simulink model "usato"  (R2016a)
settings: Solver=ode3  StartTime=0.0  StopTime=200  FixedStep=0.1  RelTol=1e-5
values from neighbouring files (symbols this model uses):
  c = 0.1    [Script.m]
  Kd = 0.9    [Script.m]
  Ki = 0.036    [Script.m]
  Kp = 0.37    [Script.m]
  N = 5    [Script.m]
libraries: simulink x2
(part 2 of 2)

== matlab function usato/sigma2 pi5 ==
  data: qpi_d_k05 input; qpi_d_k05sigma output; C2k05 input
function qpi_d_k05sigma=sigma(qpi_d_k05,C2k05)
    if(qpi_d_k05 > C2k05)
        qpi_d_k05sigma=C2k05;
    
    else
        if(qpi_d_k05 < -C2k05)
            qpi_d_k05sigma =-C2k05;
        else
        if(qpi_d_k05 == 0)
                qpi_d_k05sigma=0;
        else
            qpi_d_k05sigma=qpi_d_k05;
        end
        end
    end

== matlab function usato/sigma1 pi6 ==
  data: qpi_k02 input; qpi_k02sigma output
function qpi_k02sigma=sigma(qpi_k02)
    if(qpi_k02 > 1.05)
        qpi_k02sigma=1.05;
    
    else
        if(qpi_k02 < -1.05)
            qpi_k02sigma = -1.05;
        else
        if(qpi_k02 == 0)
                qpi_k02sigma=0;
        else
            qpi_k02sigma=qpi_k02;
        end
        end
    end

== matlab function usato/sigma2 pi6 ==
  data: qpi_d_k02 input; qpi_d_k02sigma output; C2k02 input
function qpi_d_k02sigma=sigma(qpi_d_k02,C2k02)
    if(qpi_d_k02 > C2k02)
        qpi_d_k02sigma=C2k02;
    
    else
        if(qpi_d_k02 < -C2k02)
            qpi_d_k02sigma =-C2k02;
        else
        if(qpi_d_k02 == 0)
                qpi_d_k02sigma=0;
        else
            qpi_d_k02sigma=qpi_d_k02;
        end
        end
    end

== matlab function usato/sigma1 pi7 ==
  data: qpi_k075 input; qpi_k075sigma output
function qpi_k075sigma=sigma(qpi_k075)
    if(qpi_k075 > 1.05)
        qpi_k075sigma=1.05;
    
    else
        if(qpi_k075 < -1.05)
            qpi_k075sigma = -1.05;
        else
        if(qpi_k075 == 0)
                qpi_k075sigma=0;
        else
            qpi_k075sigma=qpi_k075;
        end
        end
    end

== matlab function usato/sigma2 pi7 ==
  data: qpi_d_k075 input; qpi_d_k075sigma output; C2k075 input
function qpi_d_k075sigma=sigma(qpi_d_k075,C2k075)
    if(qpi_d_k075 > C2k075)
        qpi_d_k075sigma=C2k075;
    
    else
        if(qpi_d_k075 < -C2k075)
            qpi_d_k075sigma =-C2k075;
        else
        if(qpi_d_k075 == 0)
                qpi_d_k075sigma=0;
        else
            qpi_d_k075sigma=qpi_d_k075;
        end
        end
    end

== matlab function usato/MATLAB Function6 ==
  data: qpk01 input; qpk01sigma output
function qpk01sigma=sigma(qpk01)
    if(qpk01 > 1.05)
        qpk01sigma=1.05;
    
    else
        if(qpk01 < -1.05)
            qpk01sigma = -1.05;
        else
        if(qpk01 == 0)
                qpk01sigma=0;
        else
            qpk01sigma=qpk01;
        end
        end
    end

== matlab function usato/MATLAB Function7 ==
  data: qdk01 input; qdk01sigma output; c3pk01 input
function qdk01sigma=sigma(qdk01,c3pk01)

    if(qdk01 > c3pk01)
        qdk01sigma=c3pk01;
    
    else
        if(qdk01 < -c3pk01)
            qdk01sigma = -c3pk01;
        else
        if(qdk01 == 0)
                qdk01sigma=0;
        else
            qdk01sigma=qdk01;
        end
        end
    end

== matlab function usato/MATLAB Function8 ==
  data: qik01 input; qik01sigma output; c2pk01 input
function qik01sigma=sigma(qik01,c2pk01)
    if(qik01 > c2pk01)
        qik01sigma=c2pk01;
    
    else
        if(qik01 < -c2pk01)
            qik01sigma = -c2pk01;
        else
        if(qik01 == 0)
                qik01sigma=0;
        else
            qik01sigma=qik01;
        end
        end
    end

== matlab function usato/MATLAB Function10 ==
  data: qdk02 input; qdk02sigma output; C3pk02 input
function qdk02sigma=sigma(qdk02,C3pk02)

    if(qdk02 > C3pk02)
        qdk02sigma=C3pk02;
    
    else
        if(qdk02 < -C3pk02)
            qdk02sigma = -C3pk02;
        else
        if(qdk02 == 0)
                qdk02sigma=0;
        else
            qdk02sigma=qdk02;
        end
        end
    end

== matlab function usato/MATLAB Function11 ==
  data: qik02 input; qik02sigma output; C2pk02 input
function qik02sigma=sigma(qik02,C2pk02)
    if(qik02 > C2pk02)
        qik02sigma=C2pk02;
    
    else
        if(qik02 < -C2pk02)
            qik02sigma = -C2pk02;
        else
        if(qik02 == 0)
                qik02sigma=0;
        else
            qik02sigma=qik02;
        end
        end
    end

== matlab function usato/MATLAB Function9 ==
  data: qpk02 input; qpk02sigma output
function qpk02sigma=sigma(qpk02)
    if(qpk02 > 1.05)
        qpk02sigma=1.05;
    
    else
        if(qpk02 < -1.05)
            qpk02sigma = -1.05;
        else
        if(qpk02 == 0)
                qpk02sigma=0;
        else
            qpk02sigma=qpk02;
        end
        end
    end

== matlab function usato/MATLAB Function12 ==
  data: qdk05 input; qdk05sigma output; C3pk05 input
function qdk05sigma=sigma(qdk05,C3pk05)

    if(qdk05 > C3pk05)
        qdk05sigma=C3pk05;
    
    else
        if(qdk05 < -C3pk05)
            qdk05sigma = -C3pk05;
        else
        if(qdk05 == 0)
                qdk05sigma=0;
        else
            qdk05sigma=qdk05;
        end
        end
    end

== matlab function usato/MATLAB Function13 ==
  data: qik05 input; qik05sigma output; C2pk05 input
function qik05sigma=sigma(qik05,C2pk05)
    if(qik05 > C2pk05)
        qik05sigma=C2pk05;
    
    else
        if(qik05 < -C2pk05)
            qik05sigma = -C2pk05;
        else
        if(qik05 == 0)
                qik05sigma=0;
        else
            qik05sigma=qik05;
        end
        end
    end

== matlab function usato/MATLAB Function14 ==
  data: qpk05 input; qpk05sigma output
function qpk05sigma=sigma(qpk05)
    if(qpk05 > 1.05)
        qpk05sigma=1.05;
    
    else
        if(qpk05 < -1.05)
            qpk05sigma = -1.05;
        else
        if(qpk05 == 0)
                qpk05sigma=0;
        else
            qpk05sigma=qpk05;
        end
        end
    end

== matlab function usato/MATLAB Function15 ==
  data: qdk2 input; qdk2sigma output; C3pk2 input
function qdk2sigma=sigma(qdk2,C3pk2)

    if(qdk2 > C3pk2)
        qdk2sigma=C3pk2;
    
    else
        if(qdk2 < -C3pk2)
            qdk2sigma = -C3pk2;
        else
        if(qdk2 == 0)
                qdk2sigma=0;
        else
            qdk2sigma=qdk2;
        end
        end
    end

== matlab function usato/MATLAB Function16 ==
  data: qik2 input; qik2sigma output; C2pk2 input
function qik2sigma=sigma(qik2,C2pk2)
    if(qik2 > C2pk2)
        qik2sigma=C2pk2;
    
    else
        if(qik2 < -C2pk2)
            qik2sigma = -C2pk2;
        else
        if(qik2 == 0)
                qik2sigma=0;
        else
            qik2sigma=qik2;
        end
        end
    end

== matlab function usato/MATLAB Function17 ==
  data: qpk2 input; qpk2sigma output
function qpk2sigma=sigma(qpk2)
    if(qpk2 > 1.05)
        qpk2sigma=1.05;
    
    else
        if(qpk2 < -1.05)
            qpk2sigma = -1.05;
        else
        if(qpk2 == 0)
                qpk2sigma=0;
        else
            qpk2sigma=qpk2;
        end
        end
    end

== matlab function usato/MATLAB Function18 ==
  data: qdk26 input; qdk26sigma output; C3pk26 input
function qdk26sigma=sigma(qdk26,C3pk26)

    if(qdk26 > C3pk26)
        qdk26sigma=C3pk26;
    
    else
        if(qdk26 < -C3pk26)
            qdk26sigma = -C3pk26;
        else
        if(qdk26 == 0)
                qdk26sigma=0;
        else
            qdk26sigma=qdk26;
        end
        end
    end

== matlab function usato/MATLAB Function19 ==
  data: qik26 input; qik26sigma output; C2pk26 input
function qik26sigma=sigma(qik26,C2pk26)
    if(qik26 > C2pk26)
        qik26sigma=C2pk26;
    
    else
        if(qik26 < -C2pk26)
            qik26sigma = -C2pk26;
        else
        if(qik26 == 0)
                qik26sigma=0;
        else
            qik26sigma=qik26;
        end
        end
    end

== matlab function usato/MATLAB Function20 ==
  data: qpk26 input; qpk26sigma output
function qpk26sigma=sigma(qpk26)
    if(qpk26 > 1.05)
        qpk26sigma=1.05;
    
    else
        if(qpk26 < -1.05)
            qpk26sigma = -1.05;
        else
        if(qpk26 == 0)
                qpk26sigma=0;
        else
            qpk26sigma=qpk26;
        end
        end
    end

== matlab function usato/sigma1 pd1 ==
  data: qpd01 input; qpd01sigma output
function qpd01sigma=sigma(qpd01)
    if(qpd01 > 1.05)
        qpd01sigma=1.05;
    
    else
        if(qpd01 < -1.05)
            qpd01sigma = -1.05;
        else
        if(qpd01 == 0)
                qpd01sigma=0;
        else
            qpd01sigma=qpd01;
        end
        end
    end

== matlab function usato/sigma2 pd1 ==
  data: qi01 input; qi01sigma output; C2pd01 input
function qi01sigma=sigma(qi01,C2pd01)
    if(qi01 > C2pd01)
        qi01sigma=C2pd01;
    
    else
        if(qi01 < -C2pd01)
            qi01sigma = -C2pd01;
        else
        if(qi01 == 0)
                qi01sigma=0;
        else
            qi01sigma=qi01;
        end
        end
    end

== matlab function usato/sigma1 pd2 ==
  data: qpd001 input; qpd001sigma output
function qpd001sigma=sigma(qpd001)
    if(qpd001 > 1.05)
        qpd001sigma=1.05;
    
    else
        if(qpd001 < -1.05)
            qpd001sigma = -1.05;
        else
        if(qpd001 == 0)
                qpd001sigma=0;
        else
            qpd001sigma=qpd001;
        end
        end
    end

== matlab function usato/sigma2 pd2 ==
  data: qi001 input; qi001sigma output; C2pd001 input
function qi001sigma=sigma(qi001,C2pd001)
    if(qi001 > C2pd001)
        qi001sigma=C2pd001;
    
    else
        if(qi001 < -C2pd001)
            qi001sigma = -C2pd001;
        else
        if(qi001 == 0)
                qi001sigma=0;
        else
            qi001sigma=qi001;
        end
        end
    end

== matlab function usato/sigma1 pd3 ==
  data: qpd10 input; qpd10sigma output
function qpd10sigma=sigma(qpd10)
    if(qpd10 > 1.05)
        qpd10sigma=1.05;
    
    else
        if(qpd10 < -1.05)
            qpd10sigma = -1.05;
        else
        if(qpd10 == 0)
                qpd10sigma=0;
        else
            qpd10sigma=qpd10;
        end
        end
    end

== matlab function usato/sigma2 pd3 ==
  data: qi10 input; qi10sigma output; C2pd10 input
function qi10sigma=sigma(qi10,C2pd10)
    if(qi10 > C2pd10)
        qi10sigma=C2pd10;
    
    else
        if(qi10 < -C2pd10)
            qi10sigma = -C2pd10;
        else
        if(qi10 == 0)
                qi10sigma=0;
        else
            qi10sigma=qi10;
        end
        end
    end

== matlab function usato/sigma1 pd4 ==
  data: qpd0001 input; qpd0001sigma output
function qpd0001sigma=sigma(qpd0001)
    if(qpd0001 > 1.05)
        qpd0001sigma=1.05;
    
    else
        if(qpd0001 < -1.05)
            qpd0001sigma = -1.05;
        else
        if(qpd0001 == 0)
                qpd0001sigma=0;
        else
            qpd0001sigma=qpd0001;
        end
        end
    end

== matlab function usato/sigma2 pd4 ==
  data: qi0001 input; qi0001sigma output; C2pd0001 input
function qi0001sigma=sigma(qi0001,C2pd0001)
    if(qi0001 > C2pd0001)
        qi0001sigma=C2pd0001;
    
    else
        if(qi0001 < -C2pd0001)
            qi0001sigma = -C2pd0001;
        else
        if(qi0001 == 0)
                qi0001sigma=0;
        else
            qi0001sigma=qi0001;
        end
        end
    end

== matlab function usato/sigma1 pd5 ==
  data: qpd003 input; qpd003sigma output
function qpd003sigma=sigma(qpd003)
    if(qpd003 > 1.05)
        qpd003sigma=1.05;
    
    else
        if(qpd003 < -1.05)
            qpd003sigma = -1.05;
        else
        if(qpd003 == 0)
                qpd003sigma=0;
        else
            qpd003sigma=qpd003;
        end
        end
    end

== matlab function usato/sigma2 pd5 ==
  data: qi003 input; qi003sigma output; C2pd003 input
function qi003sigma=sigma(qi003,C2pd003)
    if(qi003 > C2pd003)
        qi003sigma=C2pd003;
    
    else
        if(qi003 < -C2pd003)
            qi003sigma = -C2pd003;
        else
        if(qi003 == 0)
                qi003sigma=0;
        else
            qi003sigma=qi003;
        end
        end
    end
